simulink model "Midterm_Project1_PE_dsandykbayeva"  (R2020a)
settings: Solver=VariableStepAuto  StartTime=0.0  StopTime=0.5  RelTol=1e-3
libraries: powerlib x18, powerlib_meascontrol x4, dspstat3 x1
settings Model: Creator=danissa_s  LastModifiedBy=danissa_s

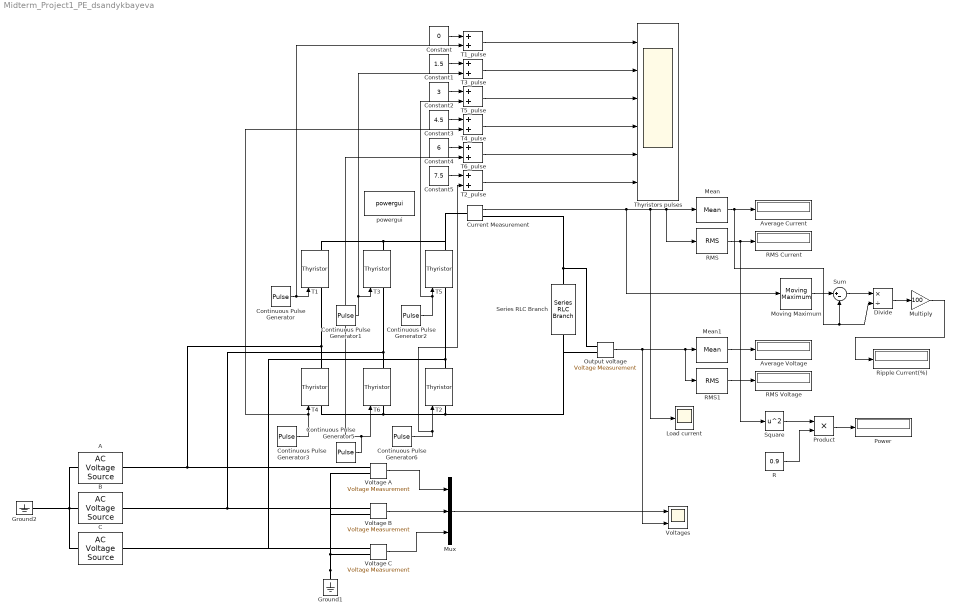
== system Midterm_Project1_PE_dsandykbayeva ==
  A : powerlib/Electrical Sources/AC Voltage Source  Amplitude=300  Phase=0  Frequency=60  SampleTime=0  Measurements=None  BusType=swing  Pref=10e3  Qref=0  Qmin=-inf  Qmax=+inf
  Average Current : Display
  Average Voltage : Display
  B : powerlib/Electrical Sources/AC Voltage Source  Amplitude=300  Phase=120  Frequency=60  SampleTime=0  Measurements=None  BusType=swing  Pref=10e3  Qref=0  Qmin=-inf  Qmax=+inf
  C : powerlib/Electrical Sources/AC Voltage Source  Amplitude=300  Phase=-120  Frequency=60  SampleTime=0  Measurements=None  BusType=swing  Pref=10e3  Qref=0  Qmin=-inf  Qmax=+inf
  Constant : Constant  Value=0
  Constant1 : Constant  Value=1.5
  Constant2 : Constant  Value=3
  Constant3 : Constant  Value=4.5
  Constant4 : Constant  Value=6
  Constant5 : Constant  Value=7.5
  Continuous Pulse Generator : DiscretePulseGenerator  PulseType=Time based  Period=1/60  PulseWidth=100/3  PhaseDelay=0.23/60
  Continuous Pulse Generator1 : DiscretePulseGenerator  PulseType=Time based  Period=1/60  PulseWidth=100/3  PhaseDelay=0.563/60
  Continuous Pulse Generator2 : DiscretePulseGenerator  PulseType=Time based  Period=1/60  PulseWidth=100/3  PhaseDelay=-0.103/60
  Continuous Pulse Generator3 : DiscretePulseGenerator  PulseType=Time based  Period=1/60  PulseWidth=100/3  PhaseDelay=0.73/60
  Continuous Pulse Generator5 : DiscretePulseGenerator  PulseType=Time based  Period=1/60  PulseWidth=100/3  PhaseDelay=0.063/60
  Continuous Pulse Generator6 : DiscretePulseGenerator  PulseType=Time based  Period=1/60  PulseWidth=100/3  PhaseDelay=0.397/60
  Current Measurement : powerlib/Measurements/Current Measurement  PhasorSimulation=off  OutputType=Complex  PSBequivalent=0
  Divide : Product  Inputs=*/
  Ground1 : powerlib/Elements/Ground  LConnTagsString=a
  Ground2 : powerlib/Elements/Ground  LConnTagsString=a
  Load current : Scope
  Mean : powerlib_meascontrol/Measurements/Mean  Freq=60  Vinit=0  Ts=0
  Mean1 : powerlib_meascontrol/Measurements/Mean  Freq=60  Vinit=0  Ts=0
  Moving Maximum : dspstat3/Moving Maximum  SpecifyWindowLength=on  WindowLength=4  SimulateUsing=Code generation
      settings: SourceProductBaseCode=DS
  Multiply : Gain  Gain=100
  Mux : Mux  Inputs=3
  Output voltage : powerlib/Measurements/Voltage Measurement  PhasorSimulation=off  OutputType=Complex  PSBequivalent=0
  Power : Display
  Product : Product
  R : Constant  Value=0.9
  RMS : powerlib_meascontrol/Measurements/RMS  TrueRMS=on  Freq=60  RMSInit=120  Ts=0
  RMS Current : Display
  RMS Voltage : Display
  RMS1 : powerlib_meascontrol/Measurements/RMS  TrueRMS=on  Freq=60  RMSInit=120  Ts=0
  Ripple Current(%) : Display
  Series RLC Branch : powerlib/Elements/Series RLC Branch  LConnTagsString=__new0  RConnTagsString=__new0  BranchType=RL  Resistance=0.9  Inductance=0.038  SetiL0=off  InitialCurrent=0  Capacitance=1e-6  Setx0=off  InitialVoltage=0  Measurements=None
  Square : Math  Operator=square  SaturateOnIntegerOverflow=on
  Sum : Sum  Inputs=|+-
  T{1..6} (6 alike) : powerlib/Power Electronics/Thyristor  Ron=0.001  Lon=0  Vf=0  IC=0  Rs=1e9  Cs=250e-9  Measurements=on
  T1_pulse : Sum
  T2_pulse : Sum
  T3_pulse : Sum
  T4_pulse : Sum
  T5_pulse : Sum
  T6_pulse : Sum
  Thyristors pulses : Scope  NumInputPorts=6
  Voltage A : powerlib/Measurements/Voltage Measurement  PhasorSimulation=off  OutputType=Complex  PSBequivalent=0
  Voltage B : powerlib/Measurements/Voltage Measurement  PhasorSimulation=off  OutputType=Complex  PSBequivalent=0
  Voltage C : powerlib/Measurements/Voltage Measurement  PhasorSimulation=off  OutputType=Complex  PSBequivalent=0
  Voltages : Scope  NumInputPorts=2
  powergui : powerlib/powergui  Priority=1  SimulationMode=Continuous  SampleTime=50e-6  frequency=60  Iterations=50  frequencyindice=60  Pbase=100e6  ErrMax=1e-4  UnitsV=kV  UnitsW=MW  buscounter=0  FunctionMessages=off  echomessages=off  EnableUseOfTLC=off  CurrentSourceSwitches=off  DisableSnubberDevices=off  DisableRonSwitches=off  DisableVfSwitches=off  DisplayEquations=off  AutomaticDiscreteSolvers=off  SolverType=Tustin/Backward Euler (TBE)  Interpol=off  ExternalGateDelay=off  methode=off  Ts=100  x0status=blocks  SPID=on  SwTol=0  HookPort=off  NonlinearTolerance=1e-4  nMaxIteration=100  ContinueOnMaxIteration=off  RestoreLinks=warning  ResistiveCurrentMeasurement=off  Frange=[0:2:500]  Ylog=off  Xlog=on  ShowGrid=off  save=off  variable=ZData  structure=0  ZoomFFT=off  StartTime=0.0  cycles=1  DisplayStyle=1  fundamental=60  FreqAxis=off  MaxFrequency=1000  frequencyindicesteady=1  RmsSteady=1  display=off
  wires:
  RMS/1 -> Square/1, RMS Current/1
  Mean/1 -> Sum/2, Divide/2, Average Current/1
  Mean1/1 -> Average Voltage/1
  Output voltage/1 -> Voltages/2, RMS1/1, Mean1/1
  RMS1/1 -> RMS Voltage/1
  Mux/1 -> Voltages/1
  Product/1 -> Power/1
  Voltage A/1 -> Mux/1
  Voltage C/1 -> Mux/3
  Voltage B/1 -> Mux/2
  Current Measurement/1 -> Moving Maximum/1, Load current/1, Mean/1, RMS/1
  Continuous Pulse Generator/1 -> T1_pulse/2, T1/1
  Continuous Pulse Generator1/1 -> T3/1, T3_pulse/2
  Continuous Pulse Generator2/1 -> T5_pulse/2, T5/1
  Continuous Pulse Generator3/1 -> T4_pulse/2, T4/1
  Continuous Pulse Generator5/1 -> T6/1, T6_pulse/2
  Continuous Pulse Generator6/1 -> T2_pulse/2, T2/1
  Constant/1 -> T1_pulse/1
  T1_pulse/1 -> Thyristors pulses/1
  T3_pulse/1 -> Thyristors pulses/2
  Constant1/1 -> T3_pulse/1
  Constant2/1 -> T5_pulse/1
  T5_pulse/1 -> Thyristors pulses/3
  Constant3/1 -> T4_pulse/1
  Constant4/1 -> T6_pulse/1
  Constant5/1 -> T2_pulse/1
  T4_pulse/1 -> Thyristors pulses/4
  T6_pulse/1 -> Thyristors pulses/5
  T2_pulse/1 -> Thyristors pulses/6
  Moving Maximum/1 -> Sum/1
  Sum/1 -> Divide/1
  Divide/1 -> Multiply/1
  Multiply/1 -> Ripple Current(%)/1
  R/1 -> Product/2
  Square/1 -> Product/1
  connections:
  T2/RConn1 -- Voltage C/LConn1 -- C/RConn1 -- T5/LConn1
  B/LConn1 -- Ground2/LConn1 -- A/LConn1 -- C/LConn1
  Ground1/LConn1 -- Voltage C/LConn2 -- Voltage A/LConn2 -- Voltage B/LConn2
  T3/RConn1 -- T1/RConn1 -- Current Measurement/LConn1 -- T5/RConn1
  Voltage B/LConn1 -- T6/RConn1 -- T3/LConn1 -- B/RConn1
  T6/LConn1 -- T4/LConn1 -- Series RLC Branch/LConn1 -- Output voltage/LConn2 -- T2/LConn1
  A/RConn1 -- T1/LConn1 -- T4/RConn1 -- Voltage A/LConn1
  Output voltage/LConn1 -- Current Measurement/RConn1 -- Series RLC Branch/RConn1
